simulink model "CAN_SDR_Model_revised"  (R2024a)
settings: Solver=VariableStepAuto  StartTime=0.0  StopTime=inf  RelTol=1e-3
undefined symbols (not defined in the file): canChannel
libraries: dspsrcs4 x7, canlib x3, canmsglib x2, commdigbbndpm3 x2, phasedtxrxlib x2, dspsigops x1, commchan3 x1
settings Model: Creator=adcli  LastModifiedBy=aceco
settings RTWCC: GPUComputeCapability=3.5

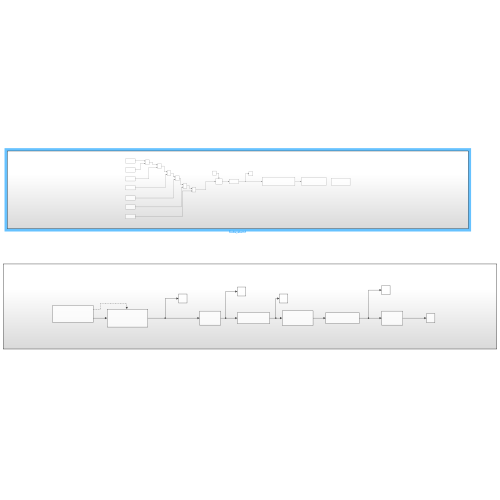
[thumbnail: Simulink's stored preview of the top-level diagram]
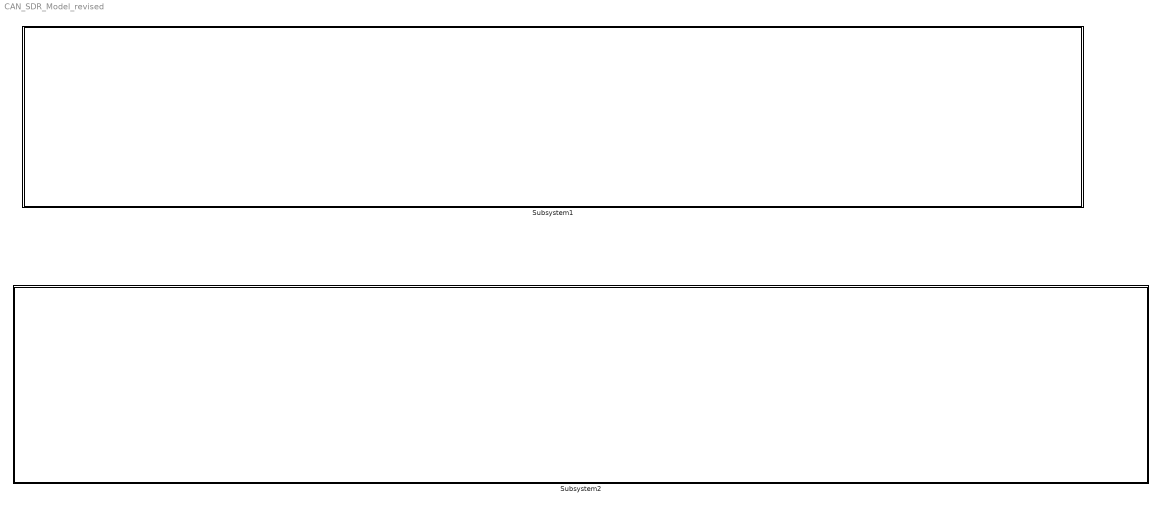
== system CAN_SDR_Model_revised ==
  Subsystem1 : Subsystem
  Subsystem2 : Subsystem

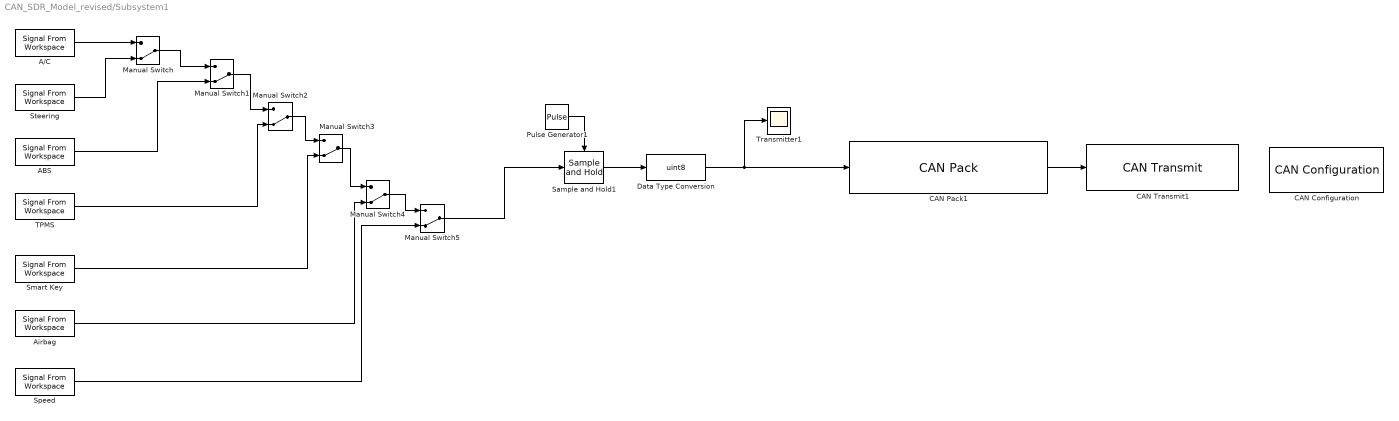
== system CAN_SDR_Model_revised/Subsystem1 ==
  A/C : dspsrcs4/Signal From Workspace  X=([0 0 0 0 1 1 1 1])  Ts=5  nsamps=1  OutputAfterFinalValue=Cyclic repetition  ignoreOrWarnInputAndFrameLengths=off  OutputFrames=off
  ABS : dspsrcs4/Signal From Workspace  X=([1 1 0 0 1 1 0 1])  Ts=5  nsamps=1  OutputAfterFinalValue=Cyclic repetition  ignoreOrWarnInputAndFrameLengths=off  OutputFrames=off
  Airbag : dspsrcs4/Signal From Workspace  X=([1 1 1 0 1 1 0 1])  Ts=5  nsamps=1  OutputAfterFinalValue=Cyclic repetition  ignoreOrWarnInputAndFrameLengths=off  OutputFrames=off
  CAN Configuration : canlib/CAN Configuration  BlockHandle=176.0007  Device=MathWorks Virtual 1 (Channel 1)  DeviceMenu=MathWorks Virtual 1 (Channel 1)  ObjConstructor=canChannel('MathWorks', 'Virtual 1', 1)  BusSpeed=500000  EnableBitParameters=off  AckMode=Normal
  CAN Pack1 : canmsglib/CAN Pack  MsgList=(none)  MsgName=CANMessage  MsgIDType=Standard (11-bit identifier)  MsgIdentifier=500  MsgLength=8  Remote=off  ApplyMinMax=off  BusOutput=off  SignalInfo={ 'Signal2', '0', '8', 'LE', 'signed', 'Standard', '0', '1', '0', '-Inf', 'Inf' }
      settings: LibrarySourceBlock=canlib/CAN Pack  DataFormat=raw data
  CAN Transmit1 : canlib/CAN Transmit  BlockHandle=305.0021  Device=MathWorks Virtual 1 (Channel 1)  DeviceMenu=MathWorks Virtual 1 (Channel 1)  ObjConstructor=canChannel('MathWorks', 'Virtual 1', 1)  EnableEventTransmit=on  EnablePeriodicTransmit=on  MessagePeriod=0.025
  Data Type Conversion : DataTypeConversion  OutDataTypeStr=uint8  SaturateOnIntegerOverflow=off  RndMeth=Floor
  Manual Switch{,1..5} (6 alike) : ManualSwitch  CurrentSetting=0
  Pulse Generator1 : DiscretePulseGenerator  Period=5  VectorParams1D=off
  Sample and Hold1 : dspsigops/Sample and Hold  trig=Either edge  initCond=0  latchinput=off
  Smart Key : dspsrcs4/Signal From Workspace  X=([0 0 0 0 0 1 1 1])  Ts=5  nsamps=1  OutputAfterFinalValue=Cyclic repetition  ignoreOrWarnInputAndFrameLengths=off  OutputFrames=off
  Speed : dspsrcs4/Signal From Workspace  X=([0 0 1 1 0 0 1 1])  Ts=5  nsamps=1  OutputAfterFinalValue=Cyclic repetition  ignoreOrWarnInputAndFrameLengths=off  OutputFrames=off
  Steering : dspsrcs4/Signal From Workspace  X=([1 0 0 0 1 1 0 1])  Ts=5  nsamps=1  OutputAfterFinalValue=Cyclic repetition  ignoreOrWarnInputAndFrameLengths=off  OutputFrames=off
  TPMS : dspsrcs4/Signal From Workspace  X=([0 1 0 1 0 1 0 1])  Ts=5  nsamps=1  OutputAfterFinalValue=Cyclic repetition  ignoreOrWarnInputAndFrameLengths=off  OutputFrames=off
  Transmitter1 : Scope
  wires:
  CAN Pack1/1 -> CAN Transmit1/1
  Data Type Conversion/1 -> Transmitter1/1, CAN Pack1/1
  Pulse Generator1/1 -> Sample and Hold1/Trigger
  Sample and Hold1/1 -> Data Type Conversion/1
  A/C/1 -> Manual Switch/1
  Manual Switch/1 -> Manual Switch1/1
  Manual Switch1/1 -> Manual Switch2/1
  Manual Switch2/1 -> Manual Switch3/1
  Manual Switch3/1 -> Manual Switch4/1
  Manual Switch4/1 -> Manual Switch5/1
  Steering/1 -> Manual Switch/2
  ABS/1 -> Manual Switch1/2
  TPMS/1 -> Manual Switch2/2
  Smart Key/1 -> Manual Switch3/2
  Airbag/1 -> Manual Switch4/2
  Speed/1 -> Manual Switch5/2
  Manual Switch5/1 -> Sample and Hold1/1

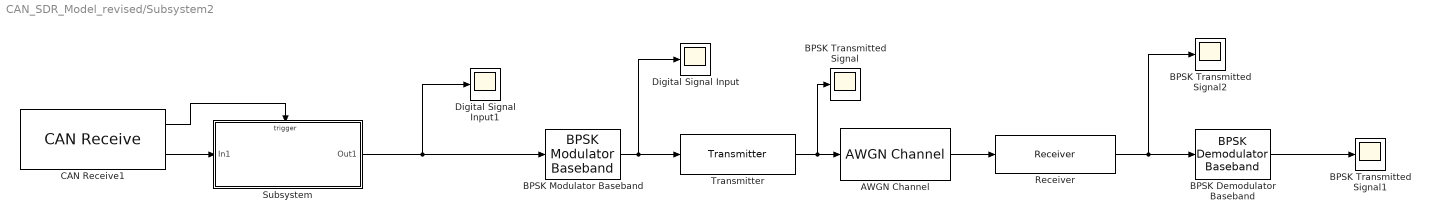
== system CAN_SDR_Model_revised/Subsystem2 ==
  AWGN Channel : commchan3/AWGN Channel  LegacyMode=off  NoiseMethod="Signal to noise ratio  (SNR)"  noiseMode="Signal to noise ratio  (SNR)"  EbNo=10  EsNo=10  SNR=-20  BitsPerSymbol=1  SignalPower=5  SamplesPerSymbol=1  SymbolPeriod=1  VarianceSource=Parameter  Variance=1  RandomStream=Global stream  Seed=67  SimulateUsing=Code generation
  BPSK Demodulator Baseband : commdigbbndpm3/BPSK Demodulator Baseband  DecType=Hard decision  VarSource=Dialog  Variance=1  Ph=pi/5  outDtype=Inherit via internal rule  derotateFactorWordLen=16  derotateFactorDataTypeStr=Inherit: Same word length as input  derotateFactorLastDataTypeStr=Inherit: Same word length as input
  BPSK Modulator Baseband : commdigbbndpm3/BPSK Modulator Baseband  Ph=-pi/5  outDtype=double  outWordLen=16  outUDDataType=sfix(16)  outFracLenMode=Best precision  outFracLen=15  outDataTypeStr=double  outLastDataTypeStr=double
  BPSK Transmitted Signal : Scope
  BPSK Transmitted Signal1 : Scope
  BPSK Transmitted Signal2 : Scope
  CAN Receive1 : canlib/CAN Receive  BlockHandle=180.0006  Device=MathWorks Virtual 1 (Channel 1)  DeviceMenu=MathWorks Virtual 1 (Channel 1)  ObjConstructor=canChannel('MathWorks', 'Virtual 1', 1)  EnableStandardIDsFilter=off  StdIDsCombo=Allow only  StandardIDs=500  EnableExtendedIDsFilter=off  ExtIDsCombo=Allow all  ExtendedIDs=0  SampleTime=.25  MsgsPerTimestep=1  InternalFilterUpdateStatus=on  BusOutput=off
  Digital Signal Input : Scope
  Digital Signal Input1 : Scope
  Receiver : phasedtxrxlib/Receiver  AddInputNoise=off  InputNoiseTemperature=290  NoiseMethod=Noise figure  NoiseFigure=3  NoiseFactor=2  NoiseTemperature=290  ReferenceTemperature=290  SampleRate=1e6  SampleRateFromInputCheckbox=off  SimulateUsing=Interpreted execution  GainMethod=Linear  Gain=20  OIP3=Inf  Table=[ -25, 5, -1; -10, 20, -2; 0, 27, 12; 5, 28, 12 ]  PhaseOffset=0  SeedSource=Auto  Seed=0
  Subsystem : Subsystem
  Transmitter : phasedtxrxlib/Transmitter  PeakPower=5000  GainMethod=Linear  Gain=20  LossFactor=0  OIP3=Inf  Table=[ -25, 5, -1; -10, 20, -2; 0, 27, 12; 5, 28, 12 ]  InUseOutputPort=off  CoherentOnTransmit=on  PhaseNoiseOutputPort=off  SimulateUsing=Interpreted execution  NoiseMethod=None  NoiseFigure=3  NoiseFactor=2  NoiseTemperature=290  ReferenceTemperature=290  SampleRate=1e6  SampleRateFromInputCheckbox=on  PhaseOffset=0  SeedSource=Auto  Seed=0
  wires:
  BPSK Modulator Baseband/1 -> Digital Signal Input/1, Transmitter/1
  BPSK Demodulator Baseband/1 -> BPSK Transmitted Signal1/1
  CAN Receive1/1 -> Subsystem/Trigger
  AWGN Channel/1 -> Receiver/1
  CAN Receive1/2 -> Subsystem/1(In1)
  Transmitter/1 -> BPSK Transmitted Signal/1, AWGN Channel/1
  Receiver/1 -> BPSK Transmitted Signal2/1, BPSK Demodulator Baseband/1
  Subsystem/1(Out1) -> Digital Signal Input1/1, BPSK Modulator Baseband/1

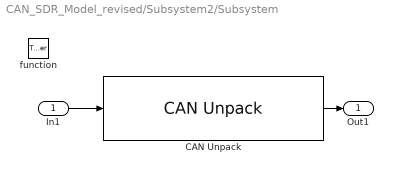
== system CAN_SDR_Model_revised/Subsystem2/Subsystem ==
  In1 : Inport
  function : TriggerPort  TriggerType=function-call  VariantControl=(inherit)
  CAN Unpack : canmsglib/CAN Unpack  MsgList=(none)  MsgName=CANMessage  MsgIDType=Standard (11-bit identifier)  MsgIdentifier=500  MsgLength=8  SignalInfo={'CANSignal','0','64','LE','double','Standard','0','1','0','-1.7e+308','1.7e+308'}  IDPort=off  TimestampPort=off  ErrorPort=off  RemotePort=off  LengthPort=off  StatusPort=off  ApplyMinMax=off
      settings: LibrarySourceBlock=canlib/CAN Unpack  DataFormat=raw data
  Out1 : Outport
  wires:
  In1/1 -> CAN Unpack/1
  CAN Unpack/1 -> Out1/1
